simulink model "SingleTrack_RTW"  (Simulink 8.7)
settings: Solver=ode1  SolverMode=SingleTasking  StartTime=0.0  StopTime=inf  FixedStep=0.001  RelTol=1e-3
PreLoadFcn:
  | vehicle = 'Car'; if ~length(which('cmcmd')), cmenv; end
  | SingleTrack_RTW_bus
  | SingleTrack_RTW_params
InitFcn:
  | vehicle = 'Car'; if ~length(which('cmcmd')), cmenv; end
  | SingleTrack_RTW_bus
undefined symbols (not defined in the file or in its folder): Car_Bdy1_mass, Car_Steering_i, Car_Whl_Radius, Car_WhlBaseF, Car_WhlBaseR, mEngineMax, PT_DL_iDiff, PT_GearBox_iForwardGears
libraries: CarMaker4SL x7
(part 1 of 3)
Description:
  | CarMaker Plug-in Model Target
settings Model: Creator=IPG  LastModifiedBy=IPG
settings DataIOCC: SignalLoggingSaveFormat=ModelDataLogs
settings OptimizationCC: ExpressionDepthLimit=2147483647
settings DebuggingCC: FcnCallInpInsideContextMsg=EnableAllAsWarning  StateNameClashWarn=warning
settings HardwareCC: TargetHWDeviceType=32-bit Generic  ProdEqTarget=off
settings RTWCC: SystemTargetFile=CarMaker.tlc  TemplateMakefile=CarMaker_unix-win64.tmf  Description=CarMaker Plug-in Model Target
settings CodeAppCC: MaxIdLength=127
settings STFCustomTargetCC: ModelReferenceCompliant=off  GeneratePreprocessorConditionals=Disable all  MultiInstanceERTCode=on  CodeInterfacePackaging=Reusable function  CPPClassGenCompliant=on  GRTInterface=off  GenerateAllocFcn=on  SystemTargetFile=CarMaker.tlc
settings GRTTargetCC: ModelReferenceCompliant=off  ParMdlRefBuildCompliant=off  CompOptLevelCompliant=off  ConcurrentExecutionCompliant=off  CombineOutputUpdateFcns=off  MatFileLogging=off  MultiInstanceERTCode=on  CodeInterfacePackaging=Reusable function  GenerateAllocFcn=on  UseToolchainInfoCompliant=off
settings CustomProperty: DataType=string  Value=..
settings EnumStrPairs: String=Car

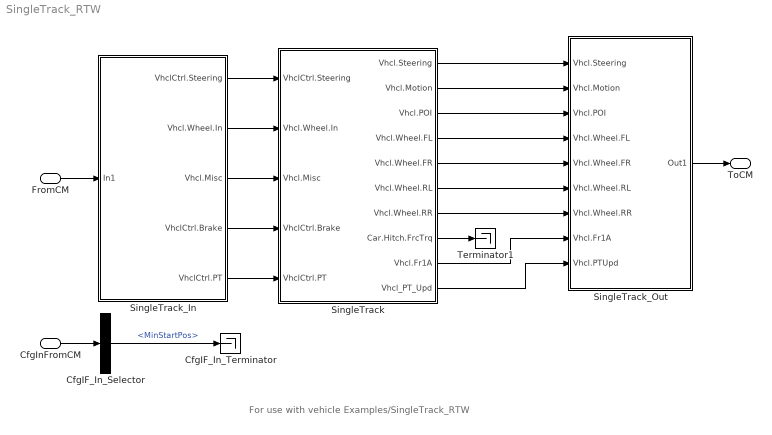
== system SingleTrack_RTW ==
  note: For use with vehicle Examples/SingleTrack_RTW
  FromCM : Inport  OutDataTypeStr=Bus: cmVehicle_CarIn
  CfgInFromCM : Inport  Port=2  OutDataTypeStr=Bus: cmVehicle_CarCfgIn
  CfgIF_In_Selector : BusSelector  OutputSignals=MinStartPos
  CfgIF_In_Terminator : Terminator
  SingleTrack : Subsystem
  SingleTrack_In : Subsystem
  SingleTrack_Out : Subsystem
  Terminator1 : Terminator
  ToCM : Outport  OutDataTypeStr=Bus: cmVehicle_CarOut
  wires:
  FromCM/1 -> SingleTrack_In/1(In1)
  CfgInFromCM/1 -> CfgIF_In_Selector/1
  CfgIF_In_Selector/1 -> CfgIF_In_Terminator/1  "<MinStartPos>"
  SingleTrack_In/1(VhclCtrl.Steering) -> SingleTrack/1(VhclCtrl.Steering)
  SingleTrack_In/2(Vhcl.Wheel.In) -> SingleTrack/2(Vhcl.Wheel.In)
  SingleTrack_In/3(Vhcl.Misc) -> SingleTrack/3(Vhcl.Misc)
  SingleTrack_In/4(VhclCtrl.Brake) -> SingleTrack/4(VhclCtrl.Brake)
  SingleTrack_In/5(VhclCtrl.PT) -> SingleTrack/5(VhclCtrl.PT)
  SingleTrack/8(Car.Hitch.FrcTrq) -> Terminator1/1
  SingleTrack/1(Vhcl.Steering) -> SingleTrack_Out/1(Vhcl.Steering)
  SingleTrack/2(Vhcl.Motion) -> SingleTrack_Out/2(Vhcl.Motion)
  SingleTrack/3(Vhcl.POI) -> SingleTrack_Out/3(Vhcl.POI)
  SingleTrack/4(Vhcl.Wheel.FL) -> SingleTrack_Out/4(Vhcl.Wheel.FL)
  SingleTrack/5(Vhcl.Wheel.FR) -> SingleTrack_Out/5(Vhcl.Wheel.FR)
  SingleTrack/6(Vhcl.Wheel.RL) -> SingleTrack_Out/6(Vhcl.Wheel.RL)
  SingleTrack/7(Vhcl.Wheel.RR) -> SingleTrack_Out/7(Vhcl.Wheel.RR)
  SingleTrack/9(Vhcl.Fr1A) -> SingleTrack_Out/8(Vhcl.Fr1A)
  SingleTrack/10(Vhcl_PT_Upd) -> SingleTrack_Out/9(Vhcl.PTUpd)
  SingleTrack_Out/1(Out1) -> ToCM/1

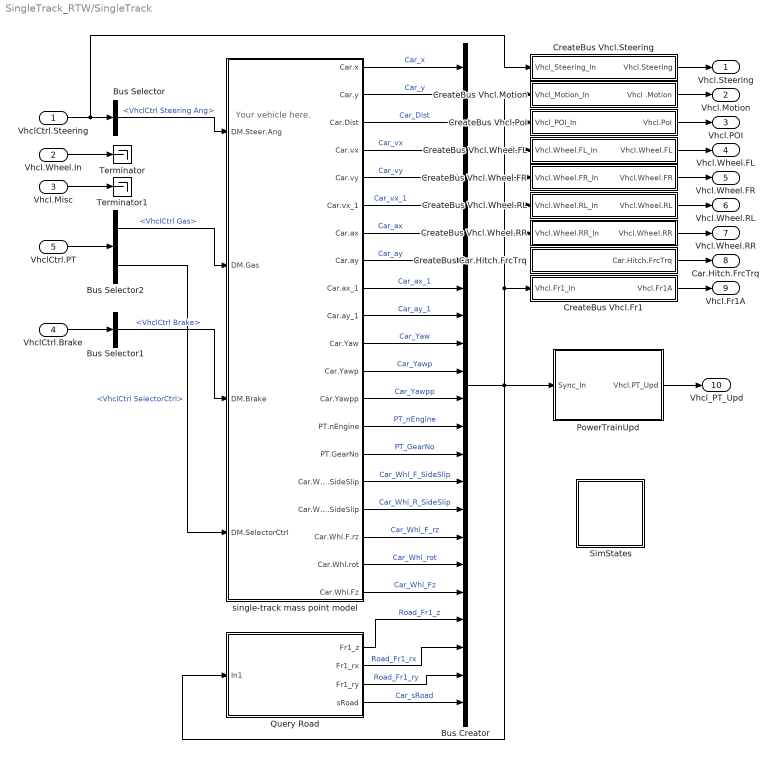
== system SingleTrack_RTW/SingleTrack ==
  note: Your vehicle here.
  VhclCtrl.Steering : Inport
  Vhcl.Wheel.In : Inport  Port=2
  Vhcl.Misc : Inport  Port=3
  VhclCtrl.Brake : Inport  Port=4
  VhclCtrl.PT : Inport  Port=5
  Bus Creator : BusCreator  Inputs=24
  Bus Selector : BusSelector  OutputSignals=VhclCtrl Steering Ang
  Bus Selector1 : BusSelector  OutputSignals=VhclCtrl Brake
  Bus Selector2 : BusSelector  OutputSignals=VhclCtrl Gas,VhclCtrl SelectorCtrl
  CreateBus Car.Hitch.FrcTrq : Subsystem
  CreateBus Vhcl.Fr1 : Subsystem
  CreateBus Vhcl.Motion : Subsystem
  CreateBus Vhcl.PoI : Subsystem
  CreateBus Vhcl.Steering : Subsystem
  CreateBus Vhcl.Wheel.FL : Subsystem
  CreateBus Vhcl.Wheel.FR : Subsystem
  CreateBus Vhcl.Wheel.RL : Subsystem
  CreateBus Vhcl.Wheel.RR : Subsystem
  PowerTrainUpd : Subsystem
  Query Road : Subsystem
  SimStates : Subsystem
  Terminator : Terminator
  Terminator1 : Terminator
  single-track mass point model : Subsystem
  Vhcl.Steering : Outport
  Vhcl.Motion : Outport  Port=2
  Vhcl.POI : Outport  Port=3
  Vhcl.Wheel.FL : Outport  Port=4
  Vhcl.Wheel.FR : Outport  Port=5
  Vhcl.Wheel.RL : Outport  Port=6
  Vhcl.Wheel.RR : Outport  Port=7
  Car.Hitch.FrcTrq : Outport  Port=8
  Vhcl.Fr1A : Outport  Port=9
  Vhcl_PT_Upd : Outport  Port=10
  wires:
  CreateBus Vhcl.Fr1/1(Vhcl.Fr1A) -> Vhcl.Fr1A/1
  single-track mass point model/20(Car.Whl.Fz) -> Bus Creator/20  "Car_Whl_Fz"
  Query Road/4(sRoad) -> Bus Creator/24  "Car_sRoad"
  CreateBus Vhcl.Motion/1(Vhcl .Motion) -> Vhcl.Motion/1
  CreateBus Vhcl.PoI/1(Vhcl.PoI) -> Vhcl.POI/1
  CreateBus Vhcl.Wheel.FL/1(Vhcl.Wheel.FL) -> Vhcl.Wheel.FL/1
  CreateBus Vhcl.Wheel.FR/1(Vhcl.Wheel.FR) -> Vhcl.Wheel.FR/1
  CreateBus Vhcl.Wheel.RL/1(Vhcl.Wheel.RL) -> Vhcl.Wheel.RL/1
  PowerTrainUpd/1(Vhcl.PT_Upd) -> Vhcl_PT_Upd/1
  Bus Selector2/1 -> single-track mass point model/2(DM.Gas)  "<VhclCtrl Gas>"
  VhclCtrl.PT/1 -> Bus Selector2/1
  VhclCtrl.Brake/1 -> Bus Selector1/1
  Query Road/3(Fr1_ry) -> Bus Creator/23  "Road_Fr1_ry"
  Query Road/2(Fr1_rx) -> Bus Creator/22  "Road_Fr1_rx"
  Query Road/1(Fr1_z) -> Bus Creator/21  "Road_Fr1_z"
  Bus Creator/1 -> CreateBus Vhcl.PoI/1(Vhcl_POI_In), CreateBus Vhcl.Wheel.FL/1(Vhcl.Wheel.FL_In), CreateBus Vhcl.Wheel.FR/1(Vhcl.Wheel.FR_In), CreateBus Vhcl.Wheel.RL/1(Vhcl.Wheel.RL_In), CreateBus Vhcl.Wheel.RR/1(Vhcl.Wheel.RR_In), Query Road/1(In1), PowerTrainUpd/1(Sync_In), CreateBus Vhcl.Motion/1(Vhcl_Motion_In), CreateBus Vhcl.Fr1/1(Vhcl.Fr1_In)
  single-track mass point model/19(Car.Whl.rot) -> Bus Creator/19  "Car_Whl_rot"
  single-track mass point model/18(Car.Whl.F.rz) -> Bus Creator/18  "Car_Whl_F_rz"
  single-track mass point model/17(Car.Whl.R.SideSlip) -> Bus Creator/17  "Car_Whl_R_SideSlip"
  single-track mass point model/16(Car.Whl.F.SideSlip) -> Bus Creator/16  "Car_Whl_F_SideSlip"
  single-track mass point model/15(PT.GearNo) -> Bus Creator/15  "PT_GearNo"
  single-track mass point model/14(PT.nEngine) -> Bus Creator/14  "PT_nEngine"
  single-track mass point model/13(Car.Yawpp) -> Bus Creator/13  "Car_Yawpp"
  single-track mass point model/12(Car.Yawp) -> Bus Creator/12  "Car_Yawp"
  single-track mass point model/11("Car.Yaw ") -> Bus Creator/11  "Car_Yaw"
  single-track mass point model/10(Car.ay_1) -> Bus Creator/10  "Car_ay_1"
  single-track mass point model/9(Car.ax_1) -> Bus Creator/9  "Car_ax_1"
  single-track mass point model/8(Car.ay) -> Bus Creator/8  "Car_ay"
  single-track mass point model/7(Car.ax) -> Bus Creator/7  "Car_ax"
  single-track mass point model/6(Car.vx_1) -> Bus Creator/6  "Car_vx_1"
  single-track mass point model/5(Car.vy) -> Bus Creator/5  "Car_vy"
  single-track mass point model/4(Car.vx) -> Bus Creator/4  "Car_vx"
  single-track mass point model/3(Car.Dist) -> Bus Creator/3  "Car_Dist"
  single-track mass point model/2(Car.y) -> Bus Creator/2  "Car_y"
  single-track mass point model/1(Car.x) -> Bus Creator/1  "Car_x"
  Bus Selector2/2 -> single-track mass point model/4(DM.SelectorCtrl)  "<VhclCtrl SelectorCtrl>"
  Bus Selector1/1 -> single-track mass point model/3(DM.Brake)  "<VhclCtrl Brake>"
  Bus Selector/1 -> single-track mass point model/1(DM.Steer.Ang)  "<VhclCtrl Steering Ang>"
  CreateBus Car.Hitch.FrcTrq/1(Car.Hitch.FrcTrq) -> Car.Hitch.FrcTrq/1
  CreateBus Vhcl.Wheel.RR/1(Vhcl.Wheel.RR) -> Vhcl.Wheel.RR/1
  CreateBus Vhcl.Steering/1(Vhcl.Steering) -> Vhcl.Steering/1
  Vhcl.Misc/1 -> Terminator1/1
  Vhcl.Wheel.In/1 -> Terminator/1
  VhclCtrl.Steering/1 -> Bus Selector/1, CreateBus Vhcl.Steering/1(Vhcl_Steering_In)

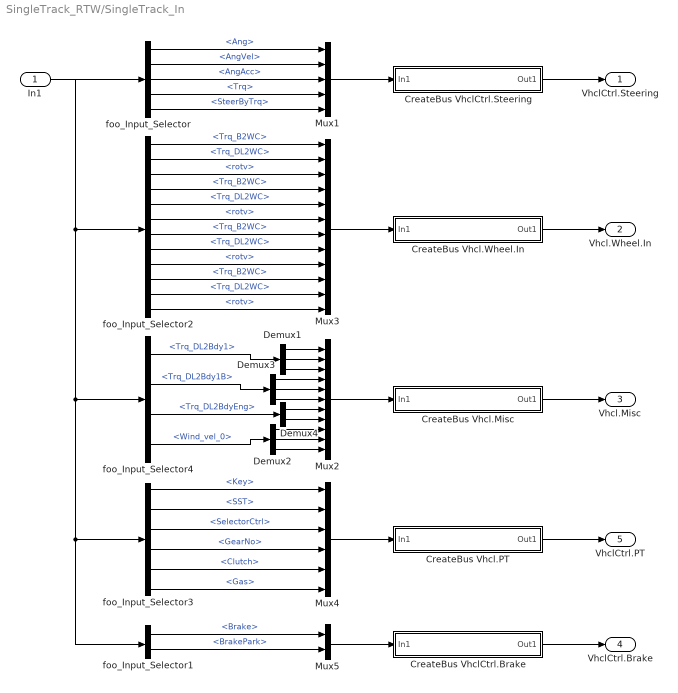
== system SingleTrack_RTW/SingleTrack_In ==
  In1 : Inport
  CreateBus Vhcl.Misc : Subsystem
  CreateBus Vhcl.PT : Subsystem
  CreateBus Vhcl.Wheel.In : Subsystem
  CreateBus VhclCtrl.Brake : Subsystem
  CreateBus VhclCtrl.Steering : Subsystem
  Demux1 : Demux  Outputs=3
  Demux2 : Demux  Outputs=3
  Demux3 : Demux  Outputs=3
  Demux4 : Demux  Outputs=2
  Mux1 : Mux  Inputs=5
  Mux2 : Mux  Inputs=11
  Mux3 : Mux  Inputs=12
  Mux4 : Mux  Inputs=6
  Mux5 : Mux  Inputs=2
  foo_Input_Selector : BusSelector  OutputSignals=VhclCtrl.Steering.Ang,VhclCtrl.Steering.AngVel,VhclCtrl.Steering.AngAcc,VhclCtrl.Steering.Trq,VhclCtrl.Steering.SteerByTrq
  foo_Input_Selector1 : BusSelector  OutputSignals=VhclCtrl.Brake,VhclCtrl.BrakePark
  foo_Input_Selector2 : BusSelector  OutputSignals=Vhcl.Wheel.FL.Trq_B2WC,Vhcl.Wheel.FL.Trq_DL2WC,Vhcl.Wheel.FL.rotv,Vhcl.Wheel.FR.Trq_B2WC,Vhcl.Wheel.FR.Trq_DL2WC,Vhcl.Wheel.FR.rotv,Vhcl.Wheel.RL.Trq_B2WC,Vhcl.Wheel.RL.Trq_DL2WC,Vhcl.Wheel.RL.rotv,Vhcl.Wheel.RR.Trq_B2WC,Vhcl.Wheel.RR.Trq_DL2WC,Vhcl.Wheel.RR.rotv
  foo_Input_Selector3 : BusSelector  OutputSignals=VhclCtrl.Key,VhclCtrl.SST,VhclCtrl.SelectorCtrl,VhclCtrl.GearNo,VhclCtrl.Clutch,VhclCtrl.Gas
  foo_Input_Selector4 : BusSelector  OutputSignals=Vhcl.Trq_DL2Bdy1,Vhcl.Trq_DL2Bdy1B,Vhcl.Trq_DL2BdyEng,Vhcl.Wind_vel_0
  VhclCtrl.Steering : Outport
  Vhcl.Wheel.In : Outport  Port=2
  Vhcl.Misc : Outport  Port=3
  VhclCtrl.Brake : Outport  Port=4
  VhclCtrl.PT : Outport  Port=5
  wires:
  foo_Input_Selector4/3 -> Demux4/1  "<Trq_DL2BdyEng>"
  Demux4/2 -> Mux2/8
  Demux4/1 -> Mux2/7
  foo_Input_Selector4/2 -> Demux3/1  "<Trq_DL2Bdy1B>"
  foo_Input_Selector4/1 -> Demux1/1  "<Trq_DL2Bdy1>"
  Demux3/3 -> Mux2/6
  Demux3/2 -> Mux2/5
  Demux3/1 -> Mux2/4
  Demux1/3 -> Mux2/3
  Demux1/2 -> Mux2/2
  Demux1/1 -> Mux2/1
  Demux2/3 -> Mux2/11
  Demux2/2 -> Mux2/10
  Demux2/1 -> Mux2/9
  foo_Input_Selector4/4 -> Demux2/1  "<Wind_vel_0>"
  foo_Input_Selector/5 -> Mux1/5  "<SteerByTrq>"
  In1/1 -> foo_Input_Selector4/1, foo_Input_Selector1/1, foo_Input_Selector3/1, foo_Input_Selector/1, foo_Input_Selector2/1
  foo_Input_Selector/1 -> Mux1/1  "<Ang>"
  foo_Input_Selector/2 -> Mux1/2  "<AngVel>"
  foo_Input_Selector/3 -> Mux1/3  "<AngAcc>"
  foo_Input_Selector/4 -> Mux1/4  "<Trq>"
  foo_Input_Selector2/1 -> Mux3/1  "<Trq_B2WC>"
  foo_Input_Selector2/2 -> Mux3/2  "<Trq_DL2WC>"
  foo_Input_Selector2/3 -> Mux3/3  "<rotv>"
  foo_Input_Selector2/4 -> Mux3/4  "<Trq_B2WC>"
  foo_Input_Selector2/5 -> Mux3/5  "<Trq_DL2WC>"
  foo_Input_Selector2/6 -> Mux3/6  "<rotv>"
  foo_Input_Selector2/7 -> Mux3/7  "<Trq_B2WC>"
  foo_Input_Selector2/8 -> Mux3/8  "<Trq_DL2WC>"
  foo_Input_Selector2/9 -> Mux3/9  "<rotv>"
  foo_Input_Selector2/10 -> Mux3/10  "<Trq_B2WC>"
  foo_Input_Selector2/11 -> Mux3/11  "<Trq_DL2WC>"
  foo_Input_Selector2/12 -> Mux3/12  "<rotv>"
  foo_Input_Selector1/1 -> Mux5/1  "<Brake>"
  Mux1/1 -> CreateBus VhclCtrl.Steering/1(In1)
  CreateBus VhclCtrl.Steering/1(Out1) -> VhclCtrl.Steering/1
  Mux3/1 -> CreateBus Vhcl.Wheel.In/1(In1)
  CreateBus Vhcl.Wheel.In/1(Out1) -> Vhcl.Wheel.In/1
  Mux2/1 -> CreateBus Vhcl.Misc/1(In1)
  CreateBus Vhcl.Misc/1(Out1) -> Vhcl.Misc/1
  Mux4/1 -> CreateBus Vhcl.PT/1(In1)
  CreateBus Vhcl.PT/1(Out1) -> VhclCtrl.PT/1
  Mux5/1 -> CreateBus VhclCtrl.Brake/1(In1)
  CreateBus VhclCtrl.Brake/1(Out1) -> VhclCtrl.Brake/1
  foo_Input_Selector1/2 -> Mux5/2  "<BrakePark>"
  foo_Input_Selector3/1 -> Mux4/1  "<Key>"
  foo_Input_Selector3/2 -> Mux4/2  "<SST>"
  foo_Input_Selector3/3 -> Mux4/3  "<SelectorCtrl>"
  foo_Input_Selector3/4 -> Mux4/4  "<GearNo>"
  foo_Input_Selector3/5 -> Mux4/5  "<Clutch>"
  foo_Input_Selector3/6 -> Mux4/6  "<Gas>"

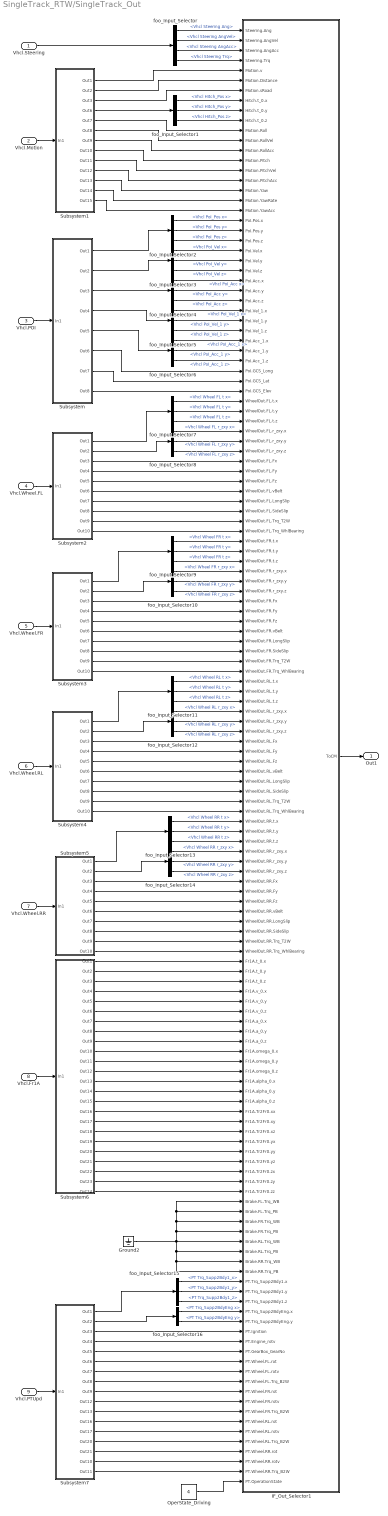
== system SingleTrack_RTW/SingleTrack_Out ==
  Vhcl.Steering : Inport
  Vhcl.Motion : Inport  Port=2
  Vhcl.POI : Inport  Port=3
  Vhcl.Wheel.FL : Inport  Port=4
  Vhcl.Wheel.FR : Inport  Port=5
  Vhcl.Wheel.RL : Inport  Port=6
  Vhcl.Wheel.RR : Inport  Port=7
  Vhcl.Fr1A : Inport  Port=8
  Vhcl.PTUpd : Inport  Port=9
  Ground2 : Ground
  IF_Out_Selector1 : Subsystem  mask(Signal Selection){}
      mask help: Signal Selection Block
      settings: OpenFcn=cmSignalSelect('SignalSelection_CB',gcb)
  OperState_Driving : Constant  Value=4
  Subsystem : Subsystem
  Subsystem1 : Subsystem
  Subsystem2 : Subsystem
  Subsystem3 : Subsystem
  Subsystem4 : Subsystem
  Subsystem5 : Subsystem
  Subsystem6 : Subsystem
  Subsystem7 : Subsystem
  foo_Input_Selector : BusSelector  OutputSignals=Vhcl Steering Ang,Vhcl Steering AngVel,Vhcl Steering AngAcc,Vhcl Steering Trq
  foo_Input_Selector1 : BusSelector  OutputSignals=Vhcl Hitch_Pos x,Vhcl Hitch_Pos y,Vhcl Hitch_Pos z
  foo_Input_Selector10 : BusSelector  OutputSignals=Vhcl Wheel FR r_zxy x,Vhcl Wheel FR r_zxy y,Vhcl Wheel FR r_zxy z
  foo_Input_Selector11 : BusSelector  OutputSignals=Vhcl Wheel RL t x,Vhcl Wheel RL t y,Vhcl Wheel RL t z
  foo_Input_Selector12 : BusSelector  OutputSignals=Vhcl Wheel RL r_zxy x,Vhcl Wheel RL r_zxy y,Vhcl Wheel RL r_zxy z
  foo_Input_Selector13 : BusSelector  OutputSignals=Vhcl Wheel RR t x,Vhcl Wheel RR t y,Vhcl Wheel RR t z
  foo_Input_Selector14 : BusSelector  OutputSignals=Vhcl Wheel RR r_zxy x,Vhcl Wheel RR r_zxy y,Vhcl Wheel RR r_zxy z
  foo_Input_Selector15 : BusSelector  OutputSignals=PT Trq_Supp2Bdy1_x,PT Trq_Supp2Bdy1_y,PT Trq_Supp2Bdy1_z
  foo_Input_Selector16 : BusSelector  OutputSignals=PT Trq_Supp2BdyEng x,PT Trq_Supp2BdyEng y
  foo_Input_Selector2 : BusSelector  OutputSignals=Vhcl PoI_Pos x,Vhcl PoI_Pos y,Vhcl PoI_Pos z
  foo_Input_Selector3 : BusSelector  OutputSignals=Vhcl PoI_Vel x,Vhcl PoI_Vel y,Vhcl PoI_Vel z
  foo_Input_Selector4 : BusSelector  OutputSignals=Vhcl PoI_Acc x,Vhcl PoI_Acc y,Vhcl PoI_Acc z
  foo_Input_Selector5 : BusSelector  OutputSignals=Vhcl PoI_Vel_1 x,Vhcl PoI_Vel_1 y,Vhcl PoI_Vel_1 z
  foo_Input_Selector6 : BusSelector  OutputSignals=Vhcl PoI_Acc_1 x,Vhcl PoI_Acc_1 y,Vhcl PoI_Acc_1 z
  foo_Input_Selector7 : BusSelector  OutputSignals=Vhcl Wheel FL t x,Vhcl Wheel FL t y,Vhcl Wheel FL t z
  foo_Input_Selector8 : BusSelector  OutputSignals=Vhcl Wheel FL r_zxy x,Vhcl Wheel FL r_zxy y,Vhcl Wheel FL r_zxy z
  foo_Input_Selector9 : BusSelector  OutputSignals=Vhcl Wheel FR t x,Vhcl Wheel FR t y,Vhcl Wheel FR t z
  Out1 : Outport
  wires:
  Subsystem1/4(Out6) -> foo_Input_Selector1/1
  Vhcl.Fr1A/1 -> Subsystem6/1(In1)
  Vhcl.Wheel.RR/1 -> Subsystem5/1(In1)
  Vhcl.Wheel.RL/1 -> Subsystem4/1(In1)
  Vhcl.Wheel.FL/1 -> Subsystem2/1(In1)
  Vhcl.POI/1 -> Subsystem/1(In1)
  Vhcl.Motion/1 -> Subsystem1/1(In1)
  Vhcl.Steering/1 -> foo_Input_Selector/1
  Vhcl.PTUpd/1 -> Subsystem7/1(In1)
  Subsystem/1(Out1) -> foo_Input_Selector2/1
  Subsystem/2(Out2) -> foo_Input_Selector3/1
  Subsystem/3(Out3) -> foo_Input_Selector4/1
  Subsystem/4(Out4) -> foo_Input_Selector5/1
  Subsystem/5(Out5) -> foo_Input_Selector6/1
  Subsystem2/1(Out1) -> foo_Input_Selector7/1
  Subsystem2/2(Out2) -> foo_Input_Selector8/1
  foo_Input_Selector15/1 -> IF_Out_Selector1/126(PT.Trq_Supp2Bdy1.x)  "<PT Trq_Supp2Bdy1_x>"
  foo_Input_Selector15/2 -> IF_Out_Selector1/127(PT.Trq_Supp2Bdy1.y)  "<PT Trq_Supp2Bdy1_y>"
  foo_Input_Selector15/3 -> IF_Out_Selector1/128(PT.Trq_Supp2Bdy1.z)  "<PT Trq_Supp2Bdy1_z>"
  foo_Input_Selector16/1 -> IF_Out_Selector1/129(PT.Trq_Supp2BdyEng.x)  "<PT Trq_Supp2BdyEng x>"
  foo_Input_Selector16/2 -> IF_Out_Selector1/130(PT.Trq_Supp2BdyEng.y)  "<PT Trq_Supp2BdyEng y>"
  Subsystem7/3(Out3) -> IF_Out_Selector1/131(PT.Ignition)
  Subsystem7/4(Out4) -> IF_Out_Selector1/132(PT.Engine_rotv)
  Subsystem7/5(Out5) -> IF_Out_Selector1/133(PT.GearBox_GearNo)
  Subsystem7/6(Out6) -> IF_Out_Selector1/134(PT.Wheel.FL.rot)
  Subsystem7/7(Out7) -> IF_Out_Selector1/135(PT.Wheel.FL.rotv)
  Subsystem7/8(Out8) -> IF_Out_Selector1/136(PT.Wheel.FL.Trq_B2W)
  Subsystem7/9(Out9) -> IF_Out_Selector1/137(PT.Wheel.FR.rot)
  Subsystem7/10(Out12) -> IF_Out_Selector1/138(PT.Wheel.FR.rotv)
  Subsystem7/11(Out13) -> IF_Out_Selector1/139(PT.Wheel.FR.Trq_B2W)
  Subsystem7/12(Out16) -> IF_Out_Selector1/140(PT.Wheel.RL.rot)
  Subsystem7/13(Out17) -> IF_Out_Selector1/141(PT.Wheel.RL.rotv)
  Subsystem7/14(Out20) -> IF_Out_Selector1/142(PT.Wheel.RL.Trq_B2W)
  Subsystem7/15(Out21) -> IF_Out_Selector1/143(PT.Wheel.RR.rot)
  Subsystem7/16(Out10) -> IF_Out_Selector1/144(PT.Wheel.RR.rotv)
  Subsystem7/17(Out11) -> IF_Out_Selector1/145(PT.Wheel.RR.Trq_B2W)
  Ground2/1 -> IF_Out_Selector1/120(Brake.FR.Trq_WB), IF_Out_Selector1/119(Brake.FL.Trq_PB), IF_Out_Selector1/118(Brake.FL.Trq_WB), IF_Out_Selector1/121(Brake.FR.Trq_PB), IF_Out_Selector1/123(Brake.RL.Trq_PB), IF_Out_Selector1/124(Brake.RR.Trq_WB), IF_Out_Selector1/125(Brake.RR.Trq_PB), IF_Out_Selector1/122(Brake.RL.Trq_WB)
  IF_Out_Selector1/1(ToCM) -> Out1/1
  OperState_Driving/1 -> IF_Out_Selector1/146(PT.OperationState)
  foo_Input_Selector/1 -> IF_Out_Selector1/1(Steering.Ang)  "<Vhcl Steering Ang>"
  foo_Input_Selector/2 -> IF_Out_Selector1/2(Steering.AngVel)  "<Vhcl Steering AngVel>"
  foo_Input_Selector/3 -> IF_Out_Selector1/3(Steering.AngAcc)  "<Vhcl Steering AngAcc>"
  foo_Input_Selector/4 -> IF_Out_Selector1/4(Steering.Trq)  "<Vhcl Steering Trq>"
  Subsystem1/1(Out1) -> IF_Out_Selector1/5(Motion.v)
  Subsystem1/2(Out2) -> IF_Out_Selector1/6(Motion.Distance)
  Subsystem1/3(Out3) -> IF_Out_Selector1/7(Motion.sRoad)
  foo_Input_Selector1/1 -> IF_Out_Selector1/8(Hitch.t_0.x)  "<Vhcl Hitch_Pos x>"
  foo_Input_Selector1/2 -> IF_Out_Selector1/9(Hitch.t_0.y)  "<Vhcl Hitch_Pos y>"
  foo_Input_Selector1/3 -> IF_Out_Selector1/10(Hitch.t_0.z)  "<Vhcl Hitch_Pos z>"
  Subsystem1/5(Out7) -> IF_Out_Selector1/11(Motion.Roll)
  Subsystem1/6(Out8) -> IF_Out_Selector1/12(Motion.RollVel)
  Subsystem1/7(Out9) -> IF_Out_Selector1/13(Motion.RollAcc)
  Subsystem1/8(Out10) -> IF_Out_Selector1/14(Motion.Pitch)
  Subsystem1/9(Out11) -> IF_Out_Selector1/15(Motion.PitchVel)
  Subsystem1/10(Out12) -> IF_Out_Selector1/16(Motion.PitchAcc)
  Subsystem1/11(Out13) -> IF_Out_Selector1/17(Motion.Yaw)
  Subsystem1/12(Out14) -> IF_Out_Selector1/18(Motion.YawRate)
  Subsystem1/13(Out15) -> IF_Out_Selector1/19(Motion.YawAcc)
  foo_Input_Selector2/1 -> IF_Out_Selector1/20(PoI.Pos.x)  "<Vhcl PoI_Pos x>"
  foo_Input_Selector2/2 -> IF_Out_Selector1/21(PoI.Pos.y)  "<Vhcl PoI_Pos y>"
  foo_Input_Selector2/3 -> IF_Out_Selector1/22(PoI.Pos.z)  "<Vhcl PoI_Pos z>"
  foo_Input_Selector3/1 -> IF_Out_Selector1/23(PoI.Vel.x)  "<Vhcl PoI_Vel x>"
  foo_Input_Selector3/2 -> IF_Out_Selector1/24(PoI.Vel.y)  "<Vhcl PoI_Vel y>"
  foo_Input_Selector3/3 -> IF_Out_Selector1/25(PoI.Vel.z)  "<Vhcl PoI_Vel z>"
  foo_Input_Selector4/1 -> IF_Out_Selector1/26(PoI.Acc.x)  "<Vhcl PoI_Acc x>"
  foo_Input_Selector4/2 -> IF_Out_Selector1/27(PoI.Acc.y)  "<Vhcl PoI_Acc y>"
  foo_Input_Selector4/3 -> IF_Out_Selector1/28(PoI.Acc.z)  "<Vhcl PoI_Acc z>"
  foo_Input_Selector5/1 -> IF_Out_Selector1/29(PoI.Vel_1.x)  "<Vhcl PoI_Vel_1 x>"
  foo_Input_Selector5/2 -> IF_Out_Selector1/30(PoI.Vel_1.y)  "<Vhcl PoI_Vel_1 y>"
  foo_Input_Selector5/3 -> IF_Out_Selector1/31(PoI.Vel_1.z)  "<Vhcl PoI_Vel_1 z>"
  foo_Input_Selector6/1 -> IF_Out_Selector1/32(PoI.Acc_1.x)  "<Vhcl PoI_Acc_1 x>"
  foo_Input_Selector6/2 -> IF_Out_Selector1/33(PoI.Acc_1.y)  "<Vhcl PoI_Acc_1 y>"
  foo_Input_Selector6/3 -> IF_Out_Selector1/34(PoI.Acc_1.z)  "<Vhcl PoI_Acc_1 z>"
  Subsystem/6(Out6) -> IF_Out_Selector1/35(PoI.GCS_Long)
  Subsystem/7(Out7) -> IF_Out_Selector1/36(PoI.GCS_Lat)
  Subsystem/8(Out8) -> IF_Out_Selector1/37(PoI.GCS_Elev)
  foo_Input_Selector7/1 -> IF_Out_Selector1/38(WheelOut.FL.t.x)  "<Vhcl Wheel FL t x>"
  foo_Input_Selector7/2 -> IF_Out_Selector1/39(WheelOut.FL.t.y)  "<Vhcl Wheel FL t y>"
  foo_Input_Selector7/3 -> IF_Out_Selector1/40(WheelOut.FL.t.z)  "<Vhcl Wheel FL t z>"
  foo_Input_Selector8/1 -> IF_Out_Selector1/41(WheelOut.FL.r_zxy.x)  "<Vhcl Wheel FL r_zxy x>"
  foo_Input_Selector8/2 -> IF_Out_Selector1/42(WheelOut.FL.r_zxy.y)  "<Vhcl Wheel FL r_zxy y>"
  foo_Input_Selector8/3 -> IF_Out_Selector1/43(WheelOut.FL.r_zxy.z)  "<Vhcl Wheel FL r_zxy z>"
  Subsystem2/3(Out3) -> IF_Out_Selector1/44(WheelOut.FL.Fx)
  Subsystem2/4(Out4) -> IF_Out_Selector1/45(WheelOut.FL.Fy)
  Subsystem2/5(Out5) -> IF_Out_Selector1/46(WheelOut.FL.Fz)
  Subsystem2/6(Out6) -> IF_Out_Selector1/47(WheelOut.FL.vBelt)
  Subsystem2/7(Out7) -> IF_Out_Selector1/48(WheelOut.FL.LongSlip)
  Subsystem2/8(Out8) -> IF_Out_Selector1/49(WheelOut.FL.SideSlip)
  Subsystem2/9(Out9) -> IF_Out_Selector1/50(WheelOut.FL.Trq_T2W)
  Subsystem2/10(Out10) -> IF_Out_Selector1/51(WheelOut.FL.Trq_WhlBearing)
  foo_Input_Selector9/1 -> IF_Out_Selector1/52(WheelOut.FR.t.x)  "<Vhcl Wheel FR t x>"
  foo_Input_Selector9/2 -> IF_Out_Selector1/53(WheelOut.FR.t.y)  "<Vhcl Wheel FR t y>"
  foo_Input_Selector9/3 -> IF_Out_Selector1/54(WheelOut.FR.t.z)  "<Vhcl Wheel FR t z>"
  foo_Input_Selector10/1 -> IF_Out_Selector1/55(WheelOut.FR.r_zxy.x)  "<Vhcl Wheel FR r_zxy x>"
  foo_Input_Selector10/2 -> IF_Out_Selector1/56(WheelOut.FR.r_zxy.y)  "<Vhcl Wheel FR r_zxy y>"
  foo_Input_Selector10/3 -> IF_Out_Selector1/57(WheelOut.FR.r_zxy.z)  "<Vhcl Wheel FR r_zxy z>"
  Subsystem3/3(Out3) -> IF_Out_Selector1/58(WheelOut.FR.Fx)
  Subsystem3/4(Out4) -> IF_Out_Selector1/59(WheelOut.FR.Fy)
  Subsystem3/5(Out5) -> IF_Out_Selector1/60(WheelOut.FR.Fz)
  Subsystem3/6(Out6) -> IF_Out_Selector1/61(WheelOut.FR.vBelt)
  Subsystem3/7(Out7) -> IF_Out_Selector1/62(WheelOut.FR.LongSlip)
  Subsystem3/8(Out8) -> IF_Out_Selector1/63(WheelOut.FR.SideSlip)
  Subsystem3/9(Out9) -> IF_Out_Selector1/64(WheelOut.FR.Trq_T2W)
  Subsystem3/10(Out10) -> IF_Out_Selector1/65(WheelOut.FR.Trq_WhlBearing)
  foo_Input_Selector11/1 -> IF_Out_Selector1/66(WheelOut.RL.t.x)  "<Vhcl Wheel RL t x>"
  foo_Input_Selector11/2 -> IF_Out_Selector1/67(WheelOut.RL.t.y)  "<Vhcl Wheel RL t y>"
  foo_Input_Selector11/3 -> IF_Out_Selector1/68(WheelOut.RL.t.z)  "<Vhcl Wheel RL t z>"
  foo_Input_Selector12/1 -> IF_Out_Selector1/69(WheelOut.RL.r_zxy.x)  "<Vhcl Wheel RL r_zxy x>"
  foo_Input_Selector12/2 -> IF_Out_Selector1/70(WheelOut.RL.r_zxy.y)  "<Vhcl Wheel RL r_zxy y>"
  foo_Input_Selector12/3 -> IF_Out_Selector1/71(WheelOut.RL.r_zxy.z)  "<Vhcl Wheel RL r_zxy z>"
  Subsystem4/3(Out3) -> IF_Out_Selector1/72(WheelOut.RL.Fx)
  Subsystem4/4(Out4) -> IF_Out_Selector1/73(WheelOut.RL.Fy)
  Subsystem4/5(Out5) -> IF_Out_Selector1/74(WheelOut.RL.Fz)
  Subsystem4/6(Out6) -> IF_Out_Selector1/75(WheelOut.RL.vBelt)
  Subsystem4/7(Out7) -> IF_Out_Selector1/76(WheelOut.RL.LongSlip)
  Subsystem4/8(Out8) -> IF_Out_Selector1/77(WheelOut.RL.SideSlip)
  Subsystem4/9(Out9) -> IF_Out_Selector1/78(WheelOut.RL.Trq_T2W)
  Subsystem4/10(Out10) -> IF_Out_Selector1/79(WheelOut.RL.Trq_WhlBearing)
  foo_Input_Selector13/1 -> IF_Out_Selector1/80(WheelOut.RR.t.x)  "<Vhcl Wheel RR t x>"
  foo_Input_Selector13/2 -> IF_Out_Selector1/81(WheelOut.RR.t.y)  "<Vhcl Wheel RR t y>"
  foo_Input_Selector13/3 -> IF_Out_Selector1/82(WheelOut.RR.t.z)  "<Vhcl Wheel RR t z>"
  foo_Input_Selector14/1 -> IF_Out_Selector1/83(WheelOut.RR.r_zxy.x)  "<Vhcl Wheel RR r_zxy x>"
  foo_Input_Selector14/2 -> IF_Out_Selector1/84(WheelOut.RR.r_zxy.y)  "<Vhcl Wheel RR r_zxy y>"
  foo_Input_Selector14/3 -> IF_Out_Selector1/85(WheelOut.RR.r_zxy.z)  "<Vhcl Wheel RR r_zxy z>"
  Subsystem5/3(Out3) -> IF_Out_Selector1/86(WheelOut.RR.Fx)
  Subsystem5/4(Out4) -> IF_Out_Selector1/87(WheelOut.RR.Fy)
  Subsystem5/5(Out5) -> IF_Out_Selector1/88(WheelOut.RR.Fz)
  Subsystem5/6(Out6) -> IF_Out_Selector1/89(WheelOut.RR.vBelt)
  Subsystem5/7(Out7) -> IF_Out_Selector1/90(WheelOut.RR.LongSlip)
  Subsystem5/8(Out8) -> IF_Out_Selector1/91(WheelOut.RR.SideSlip)
  Subsystem5/9(Out9) -> IF_Out_Selector1/92(WheelOut.RR.Trq_T2W)
  Subsystem5/10(Out10) -> IF_Out_Selector1/93(WheelOut.RR.Trq_WhlBearing)
  Subsystem6/1(Out1) -> IF_Out_Selector1/94(Fr1A.t_0.x)
  Subsystem6/2(Out2) -> IF_Out_Selector1/95(Fr1A.t_0.y)
  Subsystem6/3(Out3) -> IF_Out_Selector1/96(Fr1A.t_0.z)
  Subsystem6/4(Out4) -> IF_Out_Selector1/97(Fr1A.v_0.x)
  Subsystem6/5(Out5) -> IF_Out_Selector1/98(Fr1A.v_0.y)
  Subsystem6/6(Out6) -> IF_Out_Selector1/99(Fr1A.v_0.z)
  Subsystem6/7(Out7) -> IF_Out_Selector1/100(Fr1A.a_0.x)
  Subsystem6/8(Out8) -> IF_Out_Selector1/101(Fr1A.a_0.y)
  Subsystem6/9(Out9) -> IF_Out_Selector1/102(Fr1A.a_0.z)
  Subsystem6/10(Out10) -> IF_Out_Selector1/103(Fr1A.omega_0.x)
  Subsystem6/11(Out11) -> IF_Out_Selector1/104(Fr1A.omega_0.y)
  Subsystem6/12(Out12) -> IF_Out_Selector1/105(Fr1A.omega_0.z)
  Subsystem6/13(Out13) -> IF_Out_Selector1/106(Fr1A.alpha_0.x)
  Subsystem6/14(Out14) -> IF_Out_Selector1/107(Fr1A.alpha_0.y)
  Subsystem6/15(Out15) -> IF_Out_Selector1/108(Fr1A.alpha_0.z)
  Subsystem6/16(Out16) -> IF_Out_Selector1/109(Fr1A.Tr2Fr0.xx)
  Subsystem6/17(Out17) -> IF_Out_Selector1/110(Fr1A.Tr2Fr0.xy)
  Subsystem6/18(Out18) -> IF_Out_Selector1/111(Fr1A.Tr2Fr0.xz)
  Subsystem6/19(Out19) -> IF_Out_Selector1/112(Fr1A.Tr2Fr0.yx)
  Subsystem6/20(Out20) -> IF_Out_Selector1/113(Fr1A.Tr2Fr0.yy)
  Subsystem6/21(Out21) -> IF_Out_Selector1/114(Fr1A.Tr2Fr0.yz)
  Subsystem6/22(Out22) -> IF_Out_Selector1/115(Fr1A.Tr2Fr0.zx)
  Subsystem6/23(Out23) -> IF_Out_Selector1/116(Fr1A.Tr2Fr0.zy)
  Subsystem6/24(Out24) -> IF_Out_Selector1/117(Fr1A.Tr2Fr0.zz)
  Vhcl.Wheel.FR/1 -> Subsystem3/1(In1)
  Subsystem3/1(Out1) -> foo_Input_Selector9/1
  Subsystem3/2(Out2) -> foo_Input_Selector10/1
  Subsystem4/1(Out1) -> foo_Input_Selector11/1
  Subsystem4/2(Out2) -> foo_Input_Selector12/1
  Subsystem5/1(Out1) -> foo_Input_Selector13/1
  Subsystem5/2(Out2) -> foo_Input_Selector14/1
  Subsystem7/1(Out1) -> foo_Input_Selector15/1
  Subsystem7/2(Out2) -> foo_Input_Selector16/1

== system SingleTrack_RTW/SingleTrack/CreateBus Car.Hitch.FrcTrq ==
  Bus Creator : BusCreator  Inputs=6
  Constant{1..2,7..10} (6 alike) : Constant  Value=0
  Demux7 : Demux  Outputs=6
  Mux1 : Mux  Inputs=6
  Car.Hitch.FrcTrq : Outport
  wires:
  Demux7/1 -> Bus Creator/1  "Car Hitch Frc2Car x"
  Demux7/2 -> Bus Creator/2  "Car Hitch Frc2Car y"
  Demux7/3 -> Bus Creator/3  "Car Hitch Frc2Car z"
  Demux7/4 -> Bus Creator/4  "Car Hitch Trq2Car x"
  Demux7/5 -> Bus Creator/5  "Car Hitch Trq2Car y"
  Demux7/6 -> Bus Creator/6  "Car Hitch Trq2Car z"
  Bus Creator/1 -> Car.Hitch.FrcTrq/1
  Mux1/1 -> Demux7/1
  Constant8/1 -> Mux1/2
  Constant9/1 -> Mux1/3
  Constant10/1 -> Mux1/4
  Constant7/1 -> Mux1/1
  Constant2/1 -> Mux1/5
  Constant1/1 -> Mux1/6

== system SingleTrack_RTW/SingleTrack/CreateBus Vhcl.Fr1 ==
  Vhcl.Fr1_In : Inport
  BdyFrame2Vhcl.Fr1A : Subsystem
  Ground : Ground
  Ground1 : Ground
  Tr2Fr0 : Subsystem
  a_0 : Subsystem
  t_0 : Subsystem
  v_0 : Subsystem
  Vhcl.Fr1A : Outport
  wires:
  BdyFrame2Vhcl.Fr1A/1(Vhcl.Fr1) -> Vhcl.Fr1A/1
  Vhcl.Fr1_In/1 -> a_0/1(Car), v_0/1(Car), t_0/1(Car), Tr2Fr0/1(Car)
  Tr2Fr0/1(Tr2Fr0) -> v_0/2(Tr2Fr0), a_0/2(Tr2Fr0), BdyFrame2Vhcl.Fr1A/6(Tr2Fr0)
  t_0/1(t_0) -> BdyFrame2Vhcl.Fr1A/1(t_0)
  v_0/1(v_0) -> BdyFrame2Vhcl.Fr1A/2(v_0)
  a_0/1(a_0) -> BdyFrame2Vhcl.Fr1A/3(a_0)
  Ground1/1 -> BdyFrame2Vhcl.Fr1A/4(omega_0)
  Ground/1 -> BdyFrame2Vhcl.Fr1A/5(alpha_0)

== system SingleTrack_RTW/SingleTrack/CreateBus Vhcl.Motion ==
  Vhcl_Motion_In : Inport
  Bus Creator : BusCreator  Inputs=19
  Bus Selector : BusSelector  OutputSignals=Car_vx_1,Car_Dist,Car_sRoad,Car_x,Car_y,Road_Fr1_z,Road_Fr1_rx,Road_Fr1_ry,Car_Yaw,Car_Yawp,Car_Yawpp
  Constant{2..4,6..7,9..10} (7 alike) : Constant  Value=0
  Demux3 : Demux  Outputs=19
  Mux1 : Mux  Inputs=19
  Vhcl .Motion : Outport
  wires:
  Demux3/1 -> Bus Creator/1  "Vhcl v"
  Bus Creator/1 -> Vhcl .Motion/1
  Mux1/1 -> Demux3/1
  Demux3/2 -> Bus Creator/2  "Vhcl Distance"
  Demux3/3 -> Bus Creator/3  "Vhcl sRoad"
  Demux3/4 -> Bus Creator/4  "Vhcl sRoadAero"
  Demux3/5 -> Bus Creator/5  "Vhcl Fr1_Pos x"
  Demux3/6 -> Bus Creator/6  "Vhcl Fr1_Pos y"
  Demux3/7 -> Bus Creator/7  "Vhcl Fr1_Pos z"
  Demux3/8 -> Bus Creator/8  "Vhcl Hitch_Pos x"
  Demux3/9 -> Bus Creator/9  "Vhcl Hitch_Pos y"
  Demux3/10 -> Bus Creator/10  "Vhcl Hitch_Pos z"
  Demux3/11 -> Bus Creator/11  "Vhcl Roll"
  Demux3/12 -> Bus Creator/12  "Vhcl RollVel"
  Demux3/13 -> Bus Creator/13  "Vhcl RollAcc"
  Demux3/14 -> Bus Creator/14  "Vhcl Pitch"
  Demux3/15 -> Bus Creator/15  "Vhcl PitchVel"
  Demux3/16 -> Bus Creator/16  "Vhcl PitchAcc"
  Demux3/17 -> Bus Creator/17  "Vhcl Yaw"
  Demux3/18 -> Bus Creator/18  "Vhcl YawRate"
  Demux3/19 -> Bus Creator/19  "Vhcl YawAcc"
  Vhcl_Motion_In/1 -> Bus Selector/1
  Bus Selector/1 -> Mux1/1  "<Car_vx_1>"
  Bus Selector/2 -> Mux1/2  "<Car_Dist>"
  Bus Selector/4 -> Mux1/5  "<Car_x>"
  Bus Selector/5 -> Mux1/6  "<Car_y>"
  Constant2/1 -> Mux1/8
  Constant3/1 -> Mux1/9
  Constant4/1 -> Mux1/10
  Constant6/1 -> Mux1/12
  Constant7/1 -> Mux1/13
  Constant9/1 -> Mux1/15
  Constant10/1 -> Mux1/16
  Bus Selector/9 -> Mux1/17  "<Car_Yaw>"
  Bus Selector/10 -> Mux1/18  "<Car_Yawp>"
  Bus Selector/11 -> Mux1/19  "<Car_Yawpp>"
  Bus Selector/6 -> Mux1/7  "<Road_Fr1_z>"
  Bus Selector/7 -> Mux1/11  "<Road_Fr1_rx>"
  Bus Selector/8 -> Mux1/14  "<Road_Fr1_ry>"
  Bus Selector/3 -> Mux1/4, Mux1/3  "<Car_sRoad>"

== system SingleTrack_RTW/SingleTrack/CreateBus Vhcl.PoI ==
  Vhcl_POI_In : Inport
  Bus Creator : BusCreator  Inputs=18
  Bus Selector : BusSelector  OutputSignals=Car_x,Car_y,Road_Fr1_z,Car_vx,Car_vy,Car_ax,Car_ay,Car_vx_1,Car_ax_1,Car_ay_1
  Constant{11..13,15..19} (8 alike) : Constant  Value=0
  Demux3 : Demux  Outputs=18
  Mux1 : Mux  Inputs=18
  Vhcl.PoI : Outport
  wires:
  Demux3/1 -> Bus Creator/1  "Vhcl PoI_Pos x"
  Bus Creator/1 -> Vhcl.PoI/1
  Demux3/2 -> Bus Creator/2  "Vhcl PoI_Pos y"
  Demux3/3 -> Bus Creator/3  "Vhcl PoI_Pos z"
  Demux3/4 -> Bus Creator/4  "Vhcl PoI_Vel x"
  Demux3/5 -> Bus Creator/5  "Vhcl PoI_Vel y"
  Demux3/6 -> Bus Creator/6  "Vhcl PoI_Vel z"
  Demux3/7 -> Bus Creator/7  "Vhcl PoI_Acc x"
  Demux3/8 -> Bus Creator/8  "Vhcl PoI_Acc y"
  Demux3/9 -> Bus Creator/9  "Vhcl PoI_Acc z"
  Demux3/10 -> Bus Creator/10  "Vhcl PoI_Vel_1 x"
  Demux3/11 -> Bus Creator/11  "Vhcl PoI_Vel_1 y"
  Demux3/12 -> Bus Creator/12  "Vhcl PoI_Vel_1 z"
  Demux3/13 -> Bus Creator/13  "Vhcl PoI_Acc_1 x"
  Demux3/14 -> Bus Creator/14  "Vhcl PoI_Acc_1 y"
  Demux3/15 -> Bus Creator/15  "Vhcl PoI_Acc_1 z"
  Demux3/16 -> Bus Creator/16  "Vhcl PoI_GCS Long"
  Demux3/17 -> Bus Creator/17  "Vhcl PoI_GCS Lat"
  Demux3/18 -> Bus Creator/18  "Vhcl PoI_GCS Elev"
  Mux1/1 -> Demux3/1
  Vhcl_POI_In/1 -> Bus Selector/1
  Constant12/1 -> Mux1/16
  Constant13/1 -> Mux1/17
  Constant11/1 -> Mux1/18
  Bus Selector/1 -> Mux1/1  "<Car_x>"
  Bus Selector/2 -> Mux1/2  "<Car_y>"
  Bus Selector/3 -> Mux1/3  "<Road_Fr1_z>"
  Bus Selector/4 -> Mux1/4  "<Car_vx>"
  Bus Selector/5 -> Mux1/5  "<Car_vy>"
  Constant15/1 -> Mux1/6
  Bus Selector/6 -> Mux1/7  "<Car_ax>"
  Constant16/1 -> Mux1/9
  Constant17/1 -> Mux1/11
  Constant18/1 -> Mux1/12
  Bus Selector/9 -> Mux1/13  "<Car_ax_1>"
  Bus Selector/10 -> Mux1/14  "<Car_ay_1>"
  Constant19/1 -> Mux1/15
  Bus Selector/7 -> Mux1/8  "<Car_ay>"
  Bus Selector/8 -> Mux1/10  "<Car_vx_1>"

== system SingleTrack_RTW/SingleTrack/CreateBus Vhcl.Steering ==
  Vhcl_Steering_In : Inport
  Bus Creator : BusCreator  Inputs=4
  Bus Selector : BusSelector  OutputSignals=VhclCtrl Steering Ang,VhclCtrl Steering AngVel,VhclCtrl Steering AngAcc,VhclCtrl Steering Trq
  Demux : Demux
  Mux1 : Mux
  Vhcl.Steering : Outport
  wires:
  Demux/4 -> Bus Creator/4  "Vhcl Steering Trq"
  Demux/2 -> Bus Creator/2  "Vhcl Steering AngVel"
  Demux/3 -> Bus Creator/3  "Vhcl Steering AngAcc"
  Demux/1 -> Bus Creator/1  "Vhcl Steering Ang"
  Bus Creator/1 -> Vhcl.Steering/1
  Vhcl_Steering_In/1 -> Bus Selector/1
  Bus Selector/1 -> Mux1/1  "<VhclCtrl Steering Ang>"
  Bus Selector/2 -> Mux1/2  "<VhclCtrl Steering AngVel>"
  Bus Selector/3 -> Mux1/3  "<VhclCtrl Steering AngAcc>"
  Bus Selector/4 -> Mux1/4  "<VhclCtrl Steering Trq>"
  Mux1/1 -> Demux/1

== system SingleTrack_RTW/SingleTrack/CreateBus Vhcl.Wheel.FL ==
  Vhcl.Wheel.FL_In : Inport
  Bus Creator : BusCreator  Inputs=14
  Bus Selector : BusSelector  OutputSignals=Car_Whl_F_rz,Car_Whl_Fz,Car_Whl_F_SideSlip
  Constant{1..6,8..12} (11 alike) : Constant  Value=0
  Demux3 : Demux  Outputs=14
  Mux1 : Mux  Inputs=14
  Vhcl.Wheel.FL : Outport
  wires:
  Demux3/1 -> Bus Creator/1  "Vhcl Wheel FL t x"
  Bus Creator/1 -> Vhcl.Wheel.FL/1
  Mux1/1 -> Demux3/1
  Demux3/2 -> Bus Creator/2  "Vhcl Wheel FL t y"
  Demux3/3 -> Bus Creator/3  "Vhcl Wheel FL t z"
  Demux3/4 -> Bus Creator/4  "Vhcl Wheel FL r_zxy x"
  Demux3/5 -> Bus Creator/5  "Vhcl Wheel FL r_zxy y"
  Demux3/6 -> Bus Creator/6  "Vhcl Wheel FL r_zxy z"
  Demux3/7 -> Bus Creator/7  "Vhcl Wheel FL Fx"
  Demux3/8 -> Bus Creator/8  "Vhcl Wheel FL Fy"
  Demux3/9 -> Bus Creator/9  "Vhcl Wheel FL Fz"
  Demux3/10 -> Bus Creator/10  "Vhcl Wheel FL vBelt"
  Demux3/11 -> Bus Creator/11  "Vhcl Wheel FL LongSlip"
  Demux3/12 -> Bus Creator/12  "Vhcl Wheel FL SideSlip"
  Demux3/13 -> Bus Creator/13  "Vhcl Wheel FL Trq_T2W"
  Demux3/14 -> Bus Creator/14  "Vhcl Wheel FL Trq_WhlBearing"
  Vhcl.Wheel.FL_In/1 -> Bus Selector/1
  Bus Selector/1 -> Mux1/6  "<Car_Whl_F_rz>"
  Constant1/1 -> Mux1/1
  Constant2/1 -> Mux1/2
  Constant3/1 -> Mux1/3
  Constant4/1 -> Mux1/4
  Constant5/1 -> Mux1/5
  Constant6/1 -> Mux1/7
  Constant8/1 -> Mux1/8
  Bus Selector/3 -> Mux1/12  "<Car_Whl_F_SideSlip>"
  Constant9/1 -> Mux1/10
  Constant10/1 -> Mux1/11
  Constant12/1 -> Mux1/13
  Constant11/1 -> Mux1/14
  Bus Selector/2 -> Mux1/9  "<Car_Whl_Fz>"

== system SingleTrack_RTW/SingleTrack/CreateBus Vhcl.Wheel.FR ==
  Vhcl.Wheel.FR_In : Inport
  Bus Creator : BusCreator  Inputs=14
  Bus Selector : BusSelector  OutputSignals=Car_Whl_F_rz,Car_Whl_Fz,Car_Whl_F_SideSlip
  Constant{1..7,9..12} (11 alike) : Constant  Value=0
  Demux3 : Demux  Outputs=14
  Mux1 : Mux  Inputs=14
  Vhcl.Wheel.FR : Outport
  wires:
  Demux3/1 -> Bus Creator/1  "Vhcl Wheel FR t x"
  Bus Creator/1 -> Vhcl.Wheel.FR/1
  Demux3/2 -> Bus Creator/2  "Vhcl Wheel FR t y"
  Demux3/3 -> Bus Creator/3  "Vhcl Wheel FR t z"
  Demux3/4 -> Bus Creator/4  "Vhcl Wheel FR r_zxy x"
  Demux3/5 -> Bus Creator/5  "Vhcl Wheel FR r_zxy y"
  Demux3/6 -> Bus Creator/6  "Vhcl Wheel FR r_zxy z"
  Demux3/7 -> Bus Creator/7  "Vhcl Wheel FR Fx"
  Demux3/8 -> Bus Creator/8  "Vhcl Wheel FR Fy"
  Demux3/9 -> Bus Creator/9  "Vhcl Wheel FR Fz"
  Demux3/10 -> Bus Creator/10  "Vhcl Wheel FR vBelt"
  Demux3/11 -> Bus Creator/11  "Vhcl Wheel FR LongSlip"
  Demux3/12 -> Bus Creator/12  "Vhcl Wheel FR SideSlip"
  Demux3/13 -> Bus Creator/13  "Vhcl Wheel FR Trq_T2W"
  Demux3/14 -> Bus Creator/14  "Vhcl Wheel FR Trq_WhlBearing"
  Mux1/1 -> Demux3/1
  Vhcl.Wheel.FR_In/1 -> Bus Selector/1
  Bus Selector/1 -> Mux1/6  "<Car_Whl_F_rz>"
  Constant1/1 -> Mux1/1
  Constant2/1 -> Mux1/2
  Constant3/1 -> Mux1/3
  Constant4/1 -> Mux1/4
  Constant5/1 -> Mux1/5
  Constant6/1 -> Mux1/7
  Constant7/1 -> Mux1/8
  Bus Selector/2 -> Mux1/9  "<Car_Whl_Fz>"
  Bus Selector/3 -> Mux1/12  "<Car_Whl_F_SideSlip>"
  Constant9/1 -> Mux1/10
  Constant10/1 -> Mux1/11
  Constant12/1 -> Mux1/13
  Constant11/1 -> Mux1/14

== system SingleTrack_RTW/SingleTrack/CreateBus Vhcl.Wheel.RL ==
  Vhcl.Wheel.RL_In : Inport
  Bus Creator : BusCreator  Inputs=14
  Bus Selector : BusSelector  OutputSignals=Car_Whl_Fz,Car_Whl_R_SideSlip
  Constant{1..7,9..13} (12 alike) : Constant  Value=0
  Demux3 : Demux  Outputs=14
  Mux1 : Mux  Inputs=14
  Vhcl.Wheel.RL : Outport
  wires:
  Demux3/1 -> Bus Creator/1  "Vhcl Wheel RL t x"
  Bus Creator/1 -> Vhcl.Wheel.RL/1
  Demux3/2 -> Bus Creator/2  "Vhcl Wheel RL t y"
  Demux3/3 -> Bus Creator/3  "Vhcl Wheel RL t z"
  Demux3/4 -> Bus Creator/4  "Vhcl Wheel RL r_zxy x"
  Demux3/5 -> Bus Creator/5  "Vhcl Wheel RL r_zxy y"
  Demux3/6 -> Bus Creator/6  "Vhcl Wheel RL r_zxy z"
  Demux3/7 -> Bus Creator/7  "Vhcl Wheel RL Fx"
  Demux3/8 -> Bus Creator/8  "Vhcl Wheel RL Fy"
  Demux3/9 -> Bus Creator/9  "Vhcl Wheel RL Fz"
  Demux3/10 -> Bus Creator/10  "Vhcl Wheel RL vBelt"
  Demux3/11 -> Bus Creator/11  "Vhcl Wheel RL LongSlip"
  Demux3/12 -> Bus Creator/12  "Vhcl Wheel RL SideSlip"
  Demux3/13 -> Bus Creator/13  "Vhcl Wheel RL Trq_T2W"
  Demux3/14 -> Bus Creator/14  "Vhcl Wheel RL Trq_WhlBearing"
  Mux1/1 -> Demux3/1
  Vhcl.Wheel.RL_In/1 -> Bus Selector/1
  Constant1/1 -> Mux1/1
  Constant2/1 -> Mux1/2
  Constant3/1 -> Mux1/3
  Constant4/1 -> Mux1/4
  Constant5/1 -> Mux1/5
  Constant6/1 -> Mux1/7
  Constant7/1 -> Mux1/8
  Bus Selector/1 -> Mux1/9  "<Car_Whl_Fz>"
  Constant9/1 -> Mux1/10
  Constant10/1 -> Mux1/11
  Constant12/1 -> Mux1/13
  Constant11/1 -> Mux1/14
  Constant13/1 -> Mux1/6
  Bus Selector/2 -> Mux1/12  "<Car_Whl_R_SideSlip>"

== system SingleTrack_RTW/SingleTrack/CreateBus Vhcl.Wheel.RR ==
  Vhcl.Wheel.RR_In : Inport
  Bus Creator : BusCreator  Inputs=14
  Bus Selector : BusSelector  OutputSignals=Car_Whl_Fz,Car_Whl_R_SideSlip
  Constant{1..7,9..13} (12 alike) : Constant  Value=0
  Demux3 : Demux  Outputs=14
  Mux1 : Mux  Inputs=14
  Vhcl.Wheel.RR : Outport
  wires:
  Demux3/1 -> Bus Creator/1  "Vhcl Wheel RR t x"
  Bus Creator/1 -> Vhcl.Wheel.RR/1
  Demux3/2 -> Bus Creator/2  "Vhcl Wheel RR t y"
  Demux3/3 -> Bus Creator/3  "Vhcl Wheel RR t z"
  Demux3/4 -> Bus Creator/4  "Vhcl Wheel RR r_zxy x"
  Demux3/5 -> Bus Creator/5  "Vhcl Wheel RR r_zxy y"
  Demux3/6 -> Bus Creator/6  "Vhcl Wheel RR r_zxy z"
  Demux3/7 -> Bus Creator/7  "Vhcl Wheel RR Fx"
  Demux3/8 -> Bus Creator/8  "Vhcl Wheel RR Fy"
  Demux3/9 -> Bus Creator/9  "Vhcl Wheel RR Fz"
  Demux3/10 -> Bus Creator/10  "Vhcl Wheel RR vBelt"
  Demux3/11 -> Bus Creator/11  "Vhcl Wheel RR LongSlip"
  Demux3/12 -> Bus Creator/12  "Vhcl Wheel RR SideSlip"
  Demux3/13 -> Bus Creator/13  "Vhcl Wheel RR Trq_T2W"
  Demux3/14 -> Bus Creator/14  "Vhcl Wheel RR Trq_WhlBearing"
  Mux1/1 -> Demux3/1
  Vhcl.Wheel.RR_In/1 -> Bus Selector/1
  Constant1/1 -> Mux1/1
  Constant2/1 -> Mux1/2
  Constant3/1 -> Mux1/3
  Constant4/1 -> Mux1/4
  Constant5/1 -> Mux1/5
  Constant6/1 -> Mux1/7
  Constant7/1 -> Mux1/8
  Bus Selector/1 -> Mux1/9  "<Car_Whl_Fz>"
  Constant9/1 -> Mux1/10
  Constant10/1 -> Mux1/11
  Constant12/1 -> Mux1/13
  Constant11/1 -> Mux1/14
  Constant13/1 -> Mux1/6
  Bus Selector/2 -> Mux1/12  "<Car_Whl_R_SideSlip>"

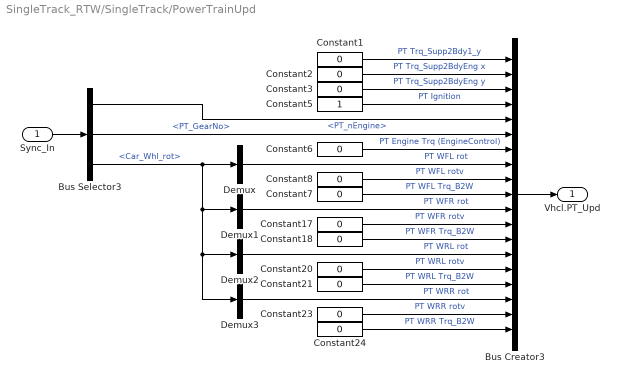
== system SingleTrack_RTW/SingleTrack/PowerTrainUpd ==
  Sync_In : Inport
  Bus Creator3 : BusCreator  Inputs=19
  Bus Selector3 : BusSelector  OutputSignals=PT_nEngine,PT_GearNo,Car_Whl_rot
  Constant{1..3,6..8,17..18,20..21,23..24} (12 alike) : Constant  Value=0
  Constant5 : Constant
  Demux{,1..3} (4 alike) : Demux  Outputs=1
  Vhcl.PT_Upd : Outport
  wires:
  Sync_In/1 -> Bus Selector3/1
  Constant1/1 -> Bus Creator3/1  "PT Trq_Supp2Bdy1_y"
  Constant2/1 -> Bus Creator3/2  "PT Trq_Supp2BdyEng x"
  Constant3/1 -> Bus Creator3/3  "PT Trq_Supp2BdyEng y"
  Constant5/1 -> Bus Creator3/4  "PT Ignition"
  Bus Selector3/1 -> Bus Creator3/5  "<PT_nEngine>"
  Constant6/1 -> Bus Creator3/7  "PT Engine Trq (EngineControl)"
  Bus Selector3/3 -> Demux2/1, Demux3/1, Demux1/1, Demux/1  "<Car_Whl_rot>"
  Constant8/1 -> Bus Creator3/9  "PT WFL rotv"
  Constant7/1 -> Bus Creator3/10  "PT WFL Trq_B2W"
  Constant17/1 -> Bus Creator3/12  "PT WFR rotv"
  Constant18/1 -> Bus Creator3/13  "PT WFR Trq_B2W"
  Constant20/1 -> Bus Creator3/15  "PT WRL rotv"
  Constant21/1 -> Bus Creator3/16  "PT WRL Trq_B2W"
  Constant23/1 -> Bus Creator3/18  "PT WRR rotv"
  Constant24/1 -> Bus Creator3/19  "PT WRR Trq_B2W"
  Bus Creator3/1 -> Vhcl.PT_Upd/1
  Demux1/1 -> Bus Creator3/11  "PT WFR rot"
  Demux2/1 -> Bus Creator3/14  "PT WRL rot"
  Demux3/1 -> Bus Creator3/17  "PT WRR rot"
  Bus Selector3/2 -> Bus Creator3/6  "<PT_GearNo>"
  Demux/1 -> Bus Creator3/8  "PT WFL rot"

== system SingleTrack_RTW/SingleTrack/Query Road ==
  In1 : Inport
  Bus Selector1 : BusSelector  OutputSignals=Car_Dist,Car_x,Car_y
  Bus Selector2 : BusSelector  OutputSignals=z,slope,grade,s
  Constant1 : Constant  Value=0
  Constant2 : Constant  Value=0
  IPGRoad5 : CarMaker4SL/IPGRoad5  xname=IPG Road  xevalmode=RouteEval XY_SZ  xconsiderbumps=off  xusepath=off  xwithcurve=off  xabort=on
  Mux : Mux  Inputs=3
  Mux1 : Mux  Inputs=2
  Read CM Parameter : CarMaker4SL/Read CM Parameter  xfile=Vehicle  xkey=Wheel.fl.pos  xnout=1  xdefaults=0  xmuxed=on
  Sum2 : Sum  SaturateOnIntegerOverflow=on  InputSameDT=on  OutDataTypeStr=Inherit: Same as first input
  Terminator : Terminator
  neg : Gain  Gain=-1  SaturateOnIntegerOverflow=on  OutDataTypeStr=Inherit: Same as input  ParamDataTypeStr=Inherit: Same as input
  Fr1_z : Outport
  Fr1_rx : Outport  Port=2
  Fr1_ry : Outport  Port=3
  sRoad : Outport  Port=4
  wires:
  Constant2/1 -> Mux/3
  Bus Selector2/2 -> Fr1_rx/1  "<slope>"
  Bus Selector2/1 -> Fr1_z/1  "<z>"
  In1/1 -> Bus Selector1/1
  Bus Selector1/3 -> Mux/2  "<Car_y>"
  Bus Selector1/2 -> Mux/1  "<Car_x>"
  Bus Selector2/3 -> neg/1  "<grade>"
  neg/1 -> Fr1_ry/1
  Bus Selector2/4 -> Sum2/1  "<s>"
  Sum2/1 -> sRoad/1
  Read CM Parameter/1 -> Sum2/2
  Mux/1 -> IPGRoad5/2
  IPGRoad5/2 -> Bus Selector2/1
  Mux1/1 -> IPGRoad5/1
  Bus Selector1/1 -> Mux1/1  "<Car_Dist>"
  Constant1/1 -> Mux1/2
  IPGRoad5/1 -> Terminator/1

== system SingleTrack_RTW/SingleTrack/SimStates ==
  note: Detect CarMaker states and transistions relevant for initialization at the start of a new testrun.
  Logical Operator : Logic  AllPortsSameDT=off  OutDataTypeStr=boolean
  Logical Operator1 : Logic  Operator=OR  AllPortsSameDT=off  OutDataTypeStr=boolean
  Memory : Memory
  Read CM Dict : CarMaker4SL/Read CM Dict  xname=SC.State  xsync=off
  Read CM Dict1 : CarMaker4SL/Read CM Dict  xname=Time  xsync=off
  Relational Operator : RelationalOperator  Operator=<=  OutDataTypeStr=boolean
  Relational Operator1 : RelationalOperator  Operator===  OutDataTypeStr=boolean
  Relational Operator2 : RelationalOperator  Operator===  OutDataTypeStr=boolean
  SCState_Simulate : Constant  Value=8
  Zero : Constant  Value=0
  detect increase : RelationalOperator  Operator=>  OutDataTypeStr=boolean
  tag scope: TRSim=global, TRStart=global
  wires:
  Read CM Dict/1 -> Relational Operator/1, Relational Operator1/2, Memory/1, detect increase/1
  SCState_Simulate/1 -> Relational Operator/2, Relational Operator1/1
  Relational Operator/1 -> Logical Operator/2
  Relational Operator1/1 -> [TRSim]
  Read CM Dict1/1 -> Relational Operator2/1
  Zero/1 -> Relational Operator2/2
  Relational Operator2/1 -> Logical Operator1/1
  Logical Operator/1 -> Logical Operator1/2
  Logical Operator1/1 -> [TRStart]
  detect increase/1 -> Logical Operator/1
  Memory/1 -> detect increase/2

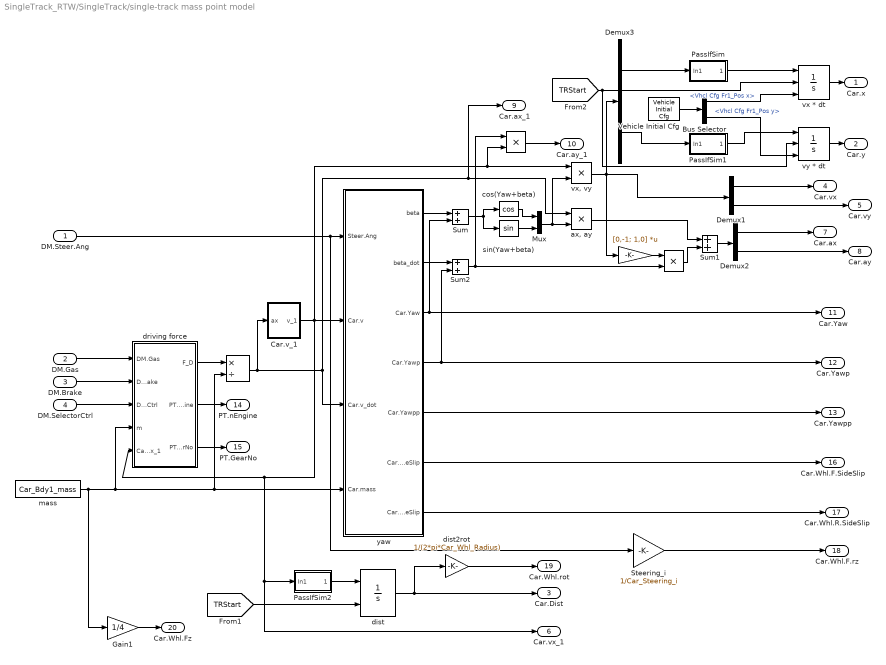
== system SingleTrack_RTW/SingleTrack/single-track mass point model ==
  DM.Steer.Ang : Inport
  DM.Gas : Inport  Port=2
  DM.Brake : Inport  Port=3
  DM.SelectorCtrl : Inport  Port=4
  " " : Gain  Gain=[0,-1; 1,0]  Multiplication=Matrix(K*u)  SaturateOnIntegerOverflow=on  OutDataTypeStr=Inherit: Same as input  ParamDataTypeStr=Inherit: Same as input
  "   " : Product  SaturateOnIntegerOverflow=on  InputSameDT=on  OutDataTypeStr=Inherit: Same as first input
  "     " : Product  SaturateOnIntegerOverflow=on  InputSameDT=on  OutDataTypeStr=Inherit: Same as first input
  "      " : Product  Inputs=*/  SaturateOnIntegerOverflow=on  InputSameDT=on  OutDataTypeStr=Inherit: Same as first input
  Bus Selector : BusSelector  OutputSignals=Vhcl Cfg Fr1_Pos x,Vhcl Cfg Fr1_Pos y
  Car.v_1 : Subsystem
  Demux1 : Demux  Outputs=2
  Demux2 : Demux  Outputs=2
  Demux3 : Demux  Outputs=2
  Gain1 : Gain  Gain=1/4
  Mux : Mux  Inputs=2
  PassIfSim : Subsystem
  PassIfSim1 : Subsystem
  PassIfSim2 : Subsystem
  "Steering_i " : Gain  Gain=1/Car_Steering_i  SaturateOnIntegerOverflow=on  OutDataTypeStr=Inherit: Same as input  ParamDataTypeStr=Inherit: Same as input
  Sum : Sum  SaturateOnIntegerOverflow=on  InputSameDT=on  OutDataTypeStr=Inherit: Same as first input
  Sum1 : Sum  SaturateOnIntegerOverflow=on  InputSameDT=on  OutDataTypeStr=Inherit: Same as first input
  Sum2 : Sum  SaturateOnIntegerOverflow=on  InputSameDT=on  OutDataTypeStr=Inherit: Same as first input
  Vehicle Initial Cfg : CarMaker4SL/Vehicle Initial Cfg
  "ax, ay" : Product  SaturateOnIntegerOverflow=on  InputSameDT=on  OutDataTypeStr=Inherit: Same as first input
  cos(Yaw+beta) : Trigonometry  Operator=cos
  dist : Integrator  ExternalReset=level
  dist2rot : Gain  Gain=1/(2*pi*Car_Whl_Radius)  SaturateOnIntegerOverflow=on  OutDataTypeStr=Inherit: Same as input  ParamDataTypeStr=Inherit: Same as input
  driving force : Subsystem
  mass : Constant  Value=Car_Bdy1_mass
  sin(Yaw+beta) : Trigonometry
  vx * dt : Integrator  ExternalReset=level  InitialConditionSource=external  InitialCondition=[0,0]
  "vx, vy" : Product  SaturateOnIntegerOverflow=on  InputSameDT=on  OutDataTypeStr=Inherit: Same as first input
  vy * dt : Integrator  ExternalReset=level  InitialConditionSource=external  InitialCondition=[0,0]
  yaw : Subsystem
  Car.x : Outport
  Car.y : Outport  Port=2
  Car.Dist : Outport  Port=3
  Car.vx : Outport  Port=4
  Car.vy : Outport  Port=5
  Car.vx_1 : Outport  Port=6
  Car.ax : Outport  Port=7
  Car.ay : Outport  Port=8
  Car.ax_1 : Outport  Port=9
  Car.ay_1 : Outport  Port=10
  "Car.Yaw " : Outport  Port=11
  Car.Yawp : Outport  Port=12
  Car.Yawpp : Outport  Port=13
  PT.nEngine : Outport  Port=14
  PT.GearNo : Outport  Port=15
  Car.Whl.F.SideSlip : Outport  Port=16
  Car.Whl.R.SideSlip : Outport  Port=17
  Car.Whl.F.rz : Outport  Port=18
  Car.Whl.rot : Outport  Port=19
  Car.Whl.Fz : Outport  Port=20
  wires:
  [TRStart] -> dist/2
  PassIfSim2/1(Out1) -> dist/1
  PassIfSim1/1(Out1) -> vy * dt/1
  Demux3/2 -> PassIfSim1/1(In1)
  PassIfSim/1(Out1) -> vx * dt/1
  Demux3/1 -> PassIfSim/1(In1)
  dist2rot/1 -> Car.Whl.rot/1
  "Steering_i "/1 -> Car.Whl.F.rz/1
  driving force/2(PT.nEngine) -> PT.nEngine/1
  mass/1 -> "      "/2, yaw/4(Car.mass), driving force/4(m), Gain1/1
  Demux1/1 -> Car.vx/1
  dist/1 -> dist2rot/1, Car.Dist/1
  Demux2/2 -> Car.ay/1
  Demux2/1 -> Car.ax/1
  Demux1/2 -> Car.vy/1
  DM.Gas/1 -> driving force/1(DM.Gas)
  DM.Brake/1 -> driving force/2(DM.Brake)
  driving force/1(F_D) -> "      "/1
  "      "/1 -> "ax, ay"/1, Car.ax_1/1, yaw/3(Car.v_dot), Car.v_1/1(ax)
  yaw/7(Car.Whl.SideSlip) -> Car.Whl.R.SideSlip/1
  yaw/6(Car.Whl.F.SideSlip) -> Car.Whl.F.SideSlip/1
  DM.Steer.Ang/1 -> "Steering_i "/1, yaw/1(Steer.Ang)
  "     "/1 -> Car.ay_1/1
  " "/1 -> "   "/1
  Sum2/1 -> "     "/1, "   "/2
  yaw/2(beta_dot) -> Sum2/1
  "ax, ay"/1 -> Sum1/1
  "   "/1 -> Sum1/2
  Sum1/1 -> Demux2/1
  Car.v_1/1(v_1) -> PassIfSim2/1(In1), Car.vx_1/1, driving force/5(Car.vx_1), "     "/2, "vx, vy"/1, yaw/2(Car.v)
  "vx, vy"/1 -> " "/1, Demux1/1, Demux3/1
  Mux/1 -> "vx, vy"/2, "ax, ay"/2
  yaw/4(Car.Yawp) -> Sum2/2, Car.Yawp/1
  yaw/5(Car.Yawpp) -> Car.Yawpp/1
  Sum/1 -> sin(Yaw+beta)/1, cos(Yaw+beta)/1
  sin(Yaw+beta)/1 -> Mux/2
  cos(Yaw+beta)/1 -> Mux/1
  yaw/3(Car.Yaw) -> "Car.Yaw "/1, Sum/2
  yaw/1(beta) -> Sum/1
  [TRStart] -> vx * dt/2, vy * dt/2
  vy * dt/1 -> Car.y/1
  vx * dt/1 -> Car.x/1
  Vehicle Initial Cfg/1 -> Bus Selector/1
  Bus Selector/2 -> vy * dt/3  "<Vhcl Cfg Fr1_Pos y>"
  Bus Selector/1 -> vx * dt/3  "<Vhcl Cfg Fr1_Pos x>"
  Gain1/1 -> Car.Whl.Fz/1
  driving force/3(PT.GearNo) -> PT.GearNo/1
  DM.SelectorCtrl/1 -> driving force/3(DM.SelectorCtrl)

== system SingleTrack_RTW/SingleTrack_In/CreateBus Vhcl.Misc ==
  In1 : Inport
  Bus Creator5 : BusCreator  Inputs=11
  Demux5 : Demux  Outputs=11
  Out1 : Outport
  wires:
  Demux5/1 -> Bus Creator5/1  "Vhcl Trq_DL2Bdy1 x"
  Demux5/2 -> Bus Creator5/2  "Vhcl Trq_DL2Bdy1 y"
  Bus Creator5/1 -> Out1/1
  In1/1 -> Demux5/1
  Demux5/3 -> Bus Creator5/3  "Vhcl Trq_DL2Bdy1 z"
  Demux5/4 -> Bus Creator5/4  "Vhcl TrqDL2Bdy1B x"
  Demux5/5 -> Bus Creator5/5  "Vhcl TrqDL2Bdy1B y"
  Demux5/6 -> Bus Creator5/6  "Vhcl TrqDL2Bdy1B z"
  Demux5/7 -> Bus Creator5/7  "Vhcl DL2BdyEng x"
  Demux5/8 -> Bus Creator5/8  "Vhcl DL2BdyEng y"
  Demux5/9 -> Bus Creator5/9  "Vhcl Wind_vel_0 x"
  Demux5/10 -> Bus Creator5/10  "Vhcl Wind_vel_0 y"
  Demux5/11 -> Bus Creator5/11  "Vhcl Wind_vel_0 z"

== system SingleTrack_RTW/SingleTrack_In/CreateBus Vhcl.PT ==
  In1 : Inport
  Bus Creator3 : BusCreator  Inputs=6
  Demux3 : Demux  Outputs=6
  Out1 : Outport
  wires:
  Demux3/6 -> Bus Creator3/6  "VhclCtrl Gas"
  Demux3/5 -> Bus Creator3/5  "VhclCtrl Clutch"
  Demux3/1 -> Bus Creator3/1  "VhclCtrl Key"
  Demux3/2 -> Bus Creator3/2  "VhclCtrl SST"
  Demux3/3 -> Bus Creator3/3  "VhclCtrl SelectorCtrl"
  Demux3/4 -> Bus Creator3/4  "VhclCtrl GearNo"
  Bus Creator3/1 -> Out1/1
  In1/1 -> Demux3/1

== system SingleTrack_RTW/SingleTrack_In/CreateBus Vhcl.Wheel.In ==
  In1 : Inport
  Bus Creator1 : BusCreator  Inputs=12
  Demux1 : Demux  Outputs=12
  Out1 : Outport
  wires:
  Demux1/1 -> Bus Creator1/1  "Vhcl Wheel FL Trq_B2WC"
  Demux1/2 -> Bus Creator1/2  "Vhcl Wheel FL Trq_DL2WC"
  Bus Creator1/1 -> Out1/1
  In1/1 -> Demux1/1
  Demux1/3 -> Bus Creator1/3  "Vhcl Wheel FL rotv"
  Demux1/4 -> Bus Creator1/4  "Vhcl Wheel FR Trq_B2WC"
  Demux1/5 -> Bus Creator1/5  "Vhcl Wheel FR Trq_DL2WC"
  Demux1/6 -> Bus Creator1/6  "Vhcl Wheel FR rotv"
  Demux1/7 -> Bus Creator1/7  "Vhcl Wheel RL Trq_B2WC"
  Demux1/8 -> Bus Creator1/8  "Vhcl Wheel RL Trq_DL2WC"
  Demux1/9 -> Bus Creator1/9  "Vhcl Wheel RL rotv"
  Demux1/10 -> Bus Creator1/10  "Vhcl Wheel RR Trq_B2WC"
  Demux1/11 -> Bus Creator1/11  "Vhcl Wheel RR Trq_DL2WC"
  Demux1/12 -> Bus Creator1/12  "Vhcl Wheel RR rotv"

== system SingleTrack_RTW/SingleTrack_In/CreateBus VhclCtrl.Brake ==
  In1 : Inport
  Bus Creator2 : BusCreator  Inputs=2
  Demux2 : Demux  Outputs=2
  Out1 : Outport
  wires:
  In1/1 -> Demux2/1
  Bus Creator2/1 -> Out1/1
  Demux2/1 -> Bus Creator2/1  "VhclCtrl Brake"
  Demux2/2 -> Bus Creator2/2  "VhclCtrl BrakePark"
